simulink model "EJ_LazoAbiertoSISO"  (R2018b)
settings: Solver=VariableStepAuto  StartTime=0.0  StopTime=4500  RelTol=1e-3  EnableMultiTasking=on
undefined symbols (not defined in the file or in its folder): sigbuilder_block
libraries: TemperatureLabLibrary x1
settings Model: Creator=johnh  LastModifiedBy=jarico
settings OptimizationCC: LifeSpan=inf
settings DebuggingCC: SFUnexpectedBacktrackingDiag=warning  SFNoUnconditionalDefaultTransitionDiag=warning  SFExecutionAtInitializationDiag=none
settings SFSimCC: SimUseLocalCustomCode=off
settings RTWCC: RTWUseLocalCustomCode=off
settings CodeAppCC: StateflowObjectComments=on
settings GRTTargetCC: TargetLangStandard=C89/C90 (ANSI)  GeneratePreprocessorConditionals=Disable all
settings ConfigComp: CovMetricSettings=dw  CovHtmlReporting=on  CovSaveCumulativeToWorkspaceVar=on  CovSaveSingleToWorkspaceVar=on  CovExternalEMLEnable=off

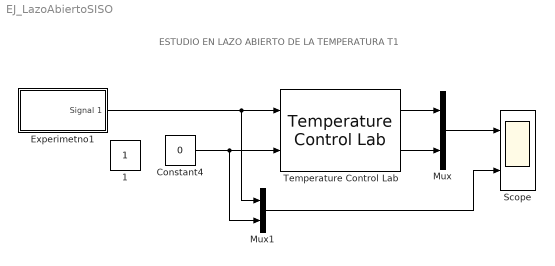
== system EJ_LazoAbiertoSISO ==
  note: ESTUDIO EN LAZO ABIERTO DE LA TEMPERATURA T1
  Constant4 : Constant  Value=0
  Experimetno1 : Subsystem  Tag=STV Subsys  LoadFcn=sigbuilder_block('load');  StartFcn=sigbuilder_block('start');  StopFcn=sigbuilder_block('stop');  ClipboardFcn=sigbuilder_block('clipboard');  mask(Sigbuilder block){tuvar=[0:10]}
      mask help: Simulink:masks:SigbuilderBlock_MD
      mask init:
      | if ~strcmp(get_param(bdroot(gcbh),'SimulationStatus'),'stopped') tuvar = sigbuilder_block('maskInit'); end
      settings: CopyFcn=sigbuilder_block('copy');  DeleteFcn=sigbuilder_block('delete');  ModelCloseFcn=sigbuilder_block('modelClose');  PreSaveFcn=sigbuilder_block('preSave');  PauseFcn=sigbuilder_block('pause');  ContinueFcn=sigbuilder_block('continue');  NameChangeFcn=sigbuilder_block('namechange');  OpenFcn=sigbuilder_block('open',[595.8 224.4 550.8 361.8 ]);  CloseFcn=sigbuilder_block('close');
      mask Display: plot(0, 0, 100, 100,[2, 2, 32, 32, 2], [68, 8, 8, 68, 68],[32, 2], [38, 38], [32, 19, 2],[53, 60, 44], [32, 17, 17, 2],[16, 16, 31, 31]);txt = getActiveGroup(gcbh);text(2, 100, txt,'verticalAlignment', 'top');
  Mux : Mux  Inputs=2
  Mux1 : Mux  Inputs=2
  Scope : Scope  NumInputPorts=2
  Temperature Control Lab : TemperatureLabLibrary/Temperature Control Lab  maxQ1=100  maxQ2=100  maxT1=80  maxT2=80  uLED=40
      settings: SourceProductName=TemperatureLabLibrary
  1 : Constant  IOType=siggen
  wires:
  Temperature Control Lab/1 -> Mux/1
  Constant4/1 -> Temperature Control Lab/2, Mux1/2
  Temperature Control Lab/2 -> Mux/2
  Mux/1 -> Scope/1
  Mux1/1 -> Scope/2
  Experimetno1/1(Signal 1) -> Temperature Control Lab/1, Mux1/1

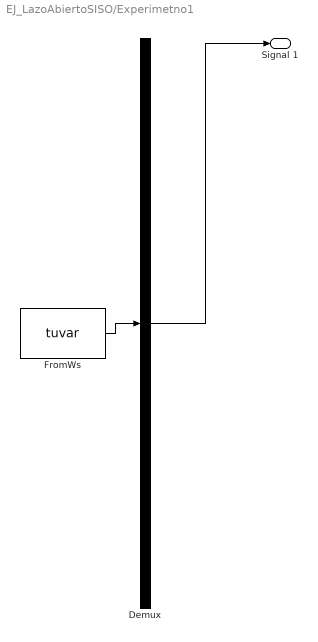
== system EJ_LazoAbiertoSISO/Experimetno1 ==
  Demux : Demux  Tag=STV Demux  Outputs=1
  FromWs : FromWorkspace  Tag=STV FromWs  VariableName=tuvar  SampleTime=0
      SigBuilderData=|
      | common.afterFinalStr = 'Extrapolate'
      | common.sampleTime = 0
      | dataSet.timeRange = [0 4500]
      | dataSet.name = 'Group 1'
      | sbobj.Groups.Name = 'Group 1'
      | sbobj.Groups.Signals.Name = 'Signal 1'
      | sbobj.Groups.Signals.XData = [0 50 50 800 800 1600 1600 2400 2400 3200 3200 4000 4000 4500]
      | sbobj.Groups.Signals.YData = [0 0 20 20 30 30 10 10 25 25 40 40 0 0]
      | sbobj.Groups.TimeRange = [0 4500]
  Signal 1 : Outport  Tag=STV Outport
  wires:
  FromWs/1 -> Demux/1
  Demux/1 -> Signal 1/1
